simulink model "sfbuilder_bususage"  (Simulink 7.6)
settings: Solver=FixedStepDiscrete  StartTime=0.0  StopTime=10.0  RelTol=1e-3
PreLoadFcn:
  | evalin('base','load sfbuilder_BusObj.mat')
settings Model: Creator=The MathWorks Inc.  SimulationMode=rapid-accelerator
settings DataIOCC: SaveState=on
settings OptimizationCC: EfficientMapNaN2IntZero=off  OptimizeModelRefInitCode=on  LifeSpan=1
settings RTWCC: SystemTargetFile=ert.tlc  TemplateMakefile=ert_default_tmf  Description=Real-Time Workshop Embedded Coder (no auto configuration)  ProcessScript=ert_make_rtw_hook
settings CodeAppCC: IgnoreCustomStorageClasses=off
settings ERTTargetCC: MultiwordLength=2048  GenerateSampleERTMain=on  ERTCustomFileTemplate=example_file_process.tlc  ConvertIfToSwitch=off

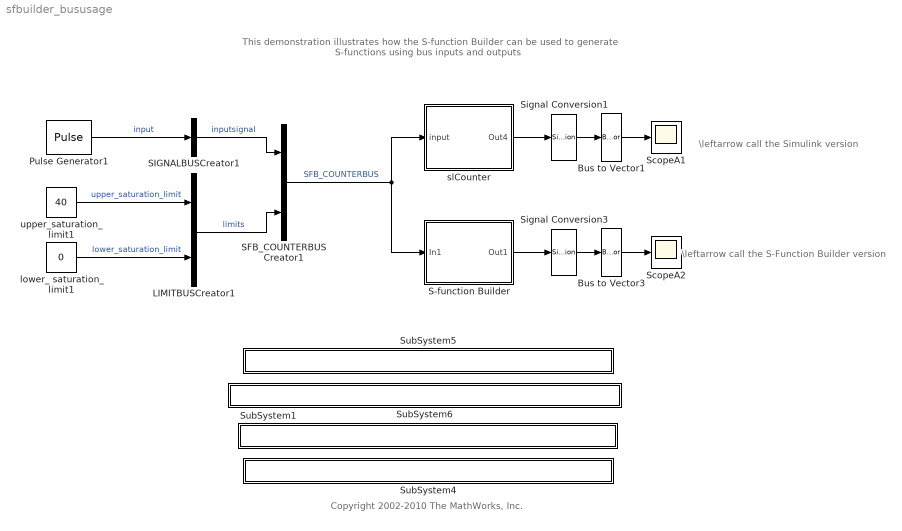
== system sfbuilder_bususage ==
  note: \leftarrow call the
      | Simulink version
  note: \leftarrow call the
      | S-Function Builder version
  note: Copyright 2002-2010 The MathWorks, Inc.
  note: This demonstration illustrates how the S-function Builder can be used to
      | generate S-functions using bus inputs and outputs
  Bus to Vector1 : BusToVector
  Bus to Vector3 : BusToVector
  LIMITBUSCreator1 : BusCreator  Inputs=2  OutDataTypeStr=Bus: SFB_LIMITBUS  NonVirtualBus=on
  Pulse Generator1 : DiscretePulseGenerator  Amplitude=int32(1)  SampleTime=0.1
  S-function Builder : Subsystem  TreatAsAtomicUnit=on
  SFB_COUNTERBUSCreator1 : BusCreator  Inputs=2  OutDataTypeStr=Bus: SFB_COUNTERBUS  NonVirtualBus=on
  SIGNALBUSCreator1 : BusCreator  Inputs=1  OutDataTypeStr=Bus: SFB_SIGNALBUS  NonVirtualBus=on
  ScopeA1 : Scope
      settings: TimeRange=30  YMax=50  SaveName=scopeout1  DataFormat=Array
  ScopeA2 : Scope
      settings: TimeRange=30  YMax=50  SaveName=scopeout2  DataFormat=Array
  Signal Conversion1 : SignalConversion  ConversionOutput=Virtual bus
  Signal Conversion3 : SignalConversion  ConversionOutput=Virtual bus
  SubSystem1 : Subsystem  mask{filename=sfbuilder_bus_bus.h}
      mask init:
      | x=sfundemo_maskdisp;
      settings: AttributesFormatString=\n  OpenFcn=sfundemo_openfcn
      mask Display: disp(x);
  SubSystem4 : Subsystem  mask{filename=sfbuilder_bus.tlc}
      mask init:
      | x=sfundemo_maskdisp;
      settings: AttributesFormatString=\n  OpenFcn=sfundemo_openfcn
      mask Display: disp(x);
  SubSystem5 : Subsystem  mask{filename=sfbuilder_bus.c}
      mask init:
      | x=sfundemo_maskdisp;
      settings: AttributesFormatString=\n  OpenFcn=sfundemo_openfcn
      mask Display: disp(x);
  SubSystem6 : Subsystem  mask{filename=sfbuilder_bus_wrapper.c}
      mask init:
      | x=sfundemo_maskdisp;
      settings: AttributesFormatString=\n  OpenFcn=sfundemo_openfcn
      mask Display: disp(x);
  lower_ saturation_ limit1 : Constant  Value=0  OutDataTypeStr=int32
  slCounter : Subsystem  TreatAsAtomicUnit=on
  upper_saturation_limit1 : Constant  Value=40  OutDataTypeStr=int32
  wires:
  upper_saturation_limit1/1 -> LIMITBUSCreator1/1  "upper_saturation_limit"
  lower_ saturation_ limit1/1 -> LIMITBUSCreator1/2  "lower_saturation_limit"
  LIMITBUSCreator1/1 -> SFB_COUNTERBUSCreator1/2  "limits"
  Pulse Generator1/1 -> SIGNALBUSCreator1/1  "input"
  SIGNALBUSCreator1/1 -> SFB_COUNTERBUSCreator1/1  "inputsignal"
  SFB_COUNTERBUSCreator1/1 -> slCounter/1(" input"), S-function Builder/1(In1)  "SFB_COUNTERBUS"
  slCounter/1(Out4) -> Signal Conversion1/1
  Signal Conversion1/1 -> Bus to Vector1/1
  Bus to Vector1/1 -> ScopeA1/1
  Signal Conversion3/1 -> Bus to Vector3/1
  Bus to Vector3/1 -> ScopeA2/1
  S-function Builder/1(Out1) -> Signal Conversion3/1

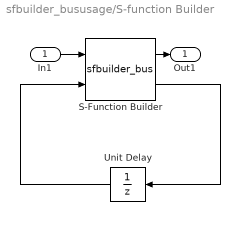
== system sfbuilder_bususage/S-function Builder ==
  In1 : Inport
  S-Function Builder : S-Function  InitFcn=try, set_param(gcb,'FunctionName','sfbuilder_bus'), end  FunctionName=sfbuilder_bus  SFunctionModules=sfbuilder_bus_wrapper  WizardData=DataTag0  EnableBusSupport=off  mask(S-Function Builder){}
      mask help: The S-Function Builder block creates a wrapper C-MEX S-function from your supplied C code with multiple input ports, output ports, and a variable number of scalar, vector, or matrix parameters. The input and output ports can propagate Simulink built-in data types, fixed-point datatypes, complex, frame, 1-D, and 2-D signals. This block also supports discrete and continuous states of type real. You can optionally have the block generate a TLC file to be used with Real-Time Workshop for code generation.
      mask init:
      | val = [[.9  0.75 0.75 1 1 .9 .9 1]',[1 1 0.75 0.75 .9 .9 1 .9]'];try , sys = get_param(gcb,'SfunBuilderFcnName');if isempty(sys), sys = get_param(gcb,'FunctionName'); end,catch, sys = get_param(gcb,'FunctionName'); end
      settings: CopyFcn=set_param(gcbh,'LinkStatus','none')  PreSaveFcn=try, set_param(gcb,'FunctionName','sfbuilder_bus'), end  OpenFcn=sfunctionwizard(gcbh)
      mask Display: plot(val(:,1),val(:,2)),disp(sys)port_label('input',1,'u0')port_label('input',2,'u1')port_label('output',1,'y0')port_label('output',2,'y1')
  Unit Delay : UnitDelay  SampleTime=-1
  Out1 : Outport
  wires:
  S-Function Builder/2 -> Unit Delay/1
  Unit Delay/1 -> S-Function Builder/2
  In1/1 -> S-Function Builder/1
  S-Function Builder/1 -> Out1/1

== system sfbuilder_bususage/SubSystem1 ==

== system sfbuilder_bususage/SubSystem4 ==

== system sfbuilder_bususage/SubSystem5 ==

== system sfbuilder_bususage/SubSystem6 ==

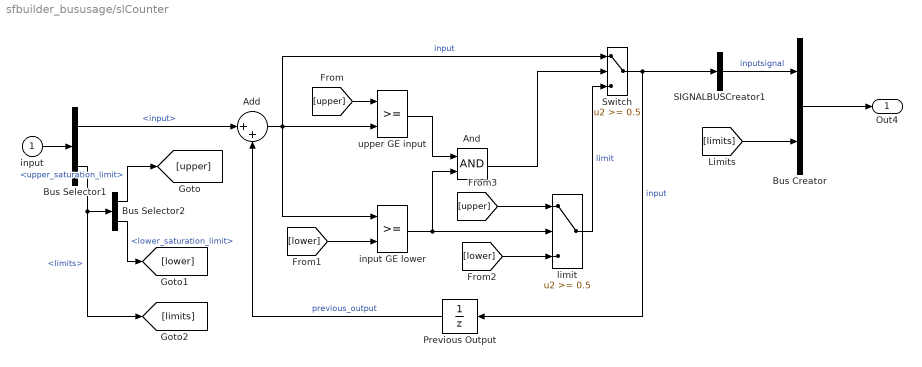
== system sfbuilder_bususage/slCounter ==
  " input" : Inport  OutDataTypeStr=Bus: SFB_COUNTERBUS
  " input GE lower" : RelationalOperator  Priority=1  InputSameDT=on
      settings: AttributesFormatString=\n
  " limit" : Switch  Threshold=0.5  SaturateOnIntegerOverflow=on  InputSameDT=on
  Add : Sum  Inputs=|++
  And : Logic
  Bus Creator : BusCreator  Inputs=2  OutDataTypeStr=Bus: SFB_COUNTERBUS  NonVirtualBus=on
  Bus Selector1 : BusSelector  OutputSignals=inputsignal.input,limits
  Bus Selector2 : BusSelector  OutputSignals=upper_saturation_limit,lower_saturation_limit
  Previous Output : UnitDelay  SampleTime=-1
  SIGNALBUSCreator1 : BusCreator  Inputs=1  OutDataTypeStr=Bus: SFB_SIGNALBUS  NonVirtualBus=on
  Switch : Switch  Threshold=0.5  SaturateOnIntegerOverflow=on  InputSameDT=on
  upper GE input : RelationalOperator  Priority=0  InputSameDT=on
      settings: AttributesFormatString=\n
  Out4 : Outport  OutDataTypeStr=Bus: SFB_COUNTERBUS
  wires:
  [upper] -> " limit"/1
  Switch/1 -> Previous Output/1, SIGNALBUSCreator1/1  "input"
  " limit"/1 -> Switch/3  "limit"
  upper GE input/1 -> And/1
  Previous Output/1 -> Add/2  "previous_output"
  [lower] -> " limit"/3
  [upper] -> upper GE input/1
  [lower] -> " input GE lower"/2
  " input GE lower"/1 -> And/2, " limit"/2
  And/1 -> Switch/2
  Add/1 -> " input GE lower"/1, upper GE input/2, Switch/1  "input"
  " input"/1 -> Bus Selector1/1
  Bus Selector1/2 -> Bus Selector2/1, [limits]  "<limits>"
  Bus Selector1/1 -> Add/1  "<input>"
  Bus Selector2/1 -> [upper]  "<upper_saturation_limit>"
  Bus Selector2/2 -> [lower]  "<lower_saturation_limit>"
  Bus Creator/1 -> Out4/1
  [limits] -> Bus Creator/2
  SIGNALBUSCreator1/1 -> Bus Creator/1  "inputsignal"
